simulink model "c28335_pmsmfoc"  (R2021b)
settings: Solver=FixedStepDiscrete  StartTime=0.0  StopTime=0.14  FixedStep=ctrlConst.TsHi  RelTol=1e-3
PreLoadFcn:
  | c28335_pmsmfoc_data
values from neighbouring files (symbols this model uses):
  ctrlConst = struct    [c28335_pmsmfoc_data.m]
  ctrlParams = tmp_P    [c28335_pmsmfoc_data.m]
undefined symbols (not defined in the file or in its folder): DiscIntNeverNeededParam, EnumControllerMode, EnumErrorType
libraries: simulink x11, slpidlib x4
(part 2 of 2)

== system c28335_pmsmfoc/Motor_Control/Field_Oriented_Controller/Current_Control/Transform_Coordinates_ABC_to_dq/Clarke_Transform ==
  note: Clarke Transform
  note: Converts balanced three-phase quantities into balanced two-phase quantities.
      | The A and B phases are converted to the direct axis (alpha) component and the quadrature axis (beta) component.
      | The alpha and beta components are still dependent on time and speed.
  phase_currents : Inport
  A_phase_current : Selector  InputPortWidth=2  IndexOptions=Index vector (dialog)  Indices=1  OutputSizes=1
  Add : Sum
  B_Gain : Gain  Gain=2
  B_phase_current : Selector  InputPortWidth=2  IndexOptions=Index vector (dialog)  Indices=2  OutputSizes=1
  Beta_Gain : Gain  Gain=1/sqrt(3)
  alpha_current : Outport
  beta_current : Outport  Port=2
  wires:
  B_phase_current/1 -> B_Gain/1
  B_Gain/1 -> Add/2
  Add/1 -> Beta_Gain/1
  Beta_Gain/1 -> beta_current/1
  phase_currents/1 -> A_phase_current/1, B_phase_current/1
  A_phase_current/1 -> Add/1, alpha_current/1

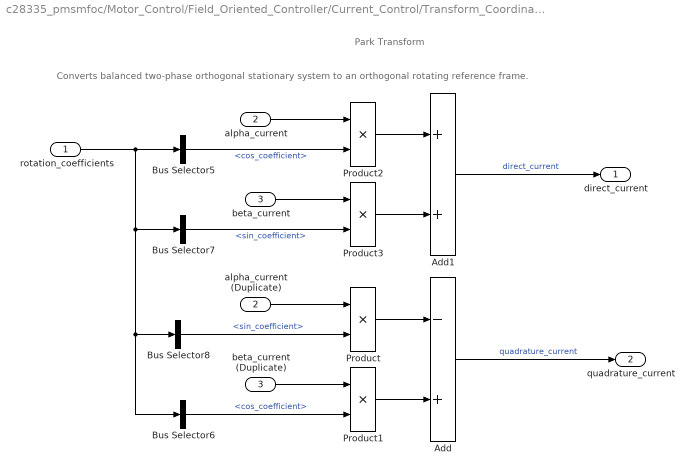
== system c28335_pmsmfoc/Motor_Control/Field_Oriented_Controller/Current_Control/Transform_Coordinates_ABC_to_dq/Park_Transform ==
  note: Park Transform
  note: Converts balanced two-phase orthogonal stationary system to an orthogonal rotating reference frame.
  rotation_coefficients : Inport
  alpha_current : Inport  Port=2
  beta_current : Inport  Port=3
  Add : Sum  Inputs=-+
  Add1 : Sum
  Bus Selector5 : BusSelector  OutputSignals=cos_coefficient
  Bus Selector6 : BusSelector  OutputSignals=cos_coefficient
  Bus Selector7 : BusSelector  OutputSignals=sin_coefficient
  Bus Selector8 : BusSelector  OutputSignals=sin_coefficient
  Product{,1..3} (4 alike) : Product  RndMeth=Zero
  alpha_current (Duplicate) : InportShadow  Port=2
  beta_current (Duplicate) : InportShadow  Port=3
  direct_current : Outport
  quadrature_current : Outport  Port=2
  wires:
  Product/1 -> Add/1
  Product1/1 -> Add/2
  Add/1 -> quadrature_current/1  "quadrature_current"
  Product2/1 -> Add1/1
  Product3/1 -> Add1/2
  Add1/1 -> direct_current/1  "direct_current"
  alpha_current (Duplicate)/1 -> Product/1
  Bus Selector8/1 -> Product/2  "<sin_coefficient>"
  Bus Selector6/1 -> Product1/2  "<cos_coefficient>"
  beta_current (Duplicate)/1 -> Product1/1
  alpha_current/1 -> Product2/1
  Bus Selector5/1 -> Product2/2  "<cos_coefficient>"
  beta_current/1 -> Product3/1
  Bus Selector7/1 -> Product3/2  "<sin_coefficient>"
  rotation_coefficients/1 -> Bus Selector5/1, Bus Selector7/1, Bus Selector8/1, Bus Selector6/1

== system c28335_pmsmfoc/Motor_Control/Field_Oriented_Controller/Current_Control/Transform_Coordinates_dq_to_ABC/Alpha_Beta_to_ABC ==
  note: 1) Only subsystems can be added as variant choices at this level
      | 2) Blocks cannot be connected at this level as connectivity is
      | automatically determined at simulation, based on the active variant
  note: Specifies which Alpha Beta to ABC coordinate transform to use.
      | The Inverse Clarke Transform is a direct sinusoidal coordinate transformation.
      | Space Vector Modulation is a technique to achieve an additional 15% increase in relative voltages between phases.
  note: Alpha Beta to ABC (Variant Subsystem)
  alpha_voltage : Inport
  beta_voltage : Inport  Port=2
  Inverse_Clarke_Transform : Subsystem  VariantControl=INVERSE_CLARKE_TRANSFORM
  Space_Vector_Modulation : Subsystem  VariantControl=SPACE_VECTOR_MODULATION
  phase_voltages : Outport

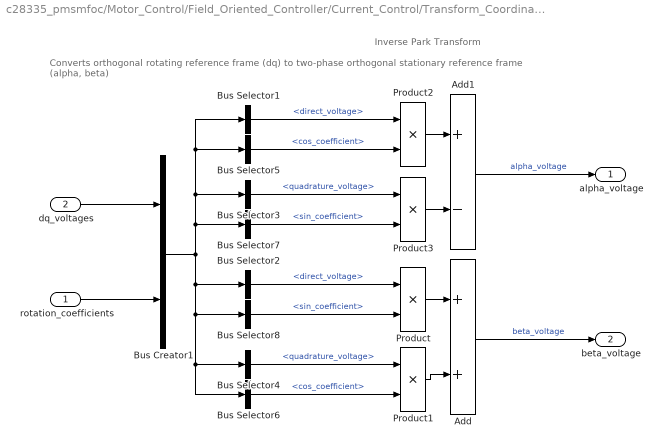
== system c28335_pmsmfoc/Motor_Control/Field_Oriented_Controller/Current_Control/Transform_Coordinates_dq_to_ABC/Inverse_Park_Transform ==
  note: Inverse Park Transform
  note: Converts orthogonal rotating reference frame (dq) to two-phase orthogonal stationary reference frame (alpha, beta)
  rotation_coefficients : Inport
  dq_voltages : Inport  Port=2
  Add : Sum
  Add1 : Sum  Inputs=+-
  Bus Creator1 : BusCreator  Inputs=2
  Bus Selector1 : BusSelector  OutputSignals=signal1.direct_voltage
  Bus Selector2 : BusSelector  OutputSignals=signal1.direct_voltage
  Bus Selector3 : BusSelector  OutputSignals=signal1.quadrature_voltage
  Bus Selector4 : BusSelector  OutputSignals=signal1.quadrature_voltage
  Bus Selector5 : BusSelector  OutputSignals=signal2.cos_coefficient
  Bus Selector6 : BusSelector  OutputSignals=signal2.cos_coefficient
  Bus Selector7 : BusSelector  OutputSignals=signal2.sin_coefficient
  Bus Selector8 : BusSelector  OutputSignals=signal2.sin_coefficient
  Product{,1..3} (4 alike) : Product  RndMeth=Zero
  alpha_voltage : Outport
  beta_voltage : Outport  Port=2
  wires:
  Product/1 -> Add/1
  Product1/1 -> Add/2
  Add/1 -> beta_voltage/1  "beta_voltage"
  Product2/1 -> Add1/1
  Product3/1 -> Add1/2
  Add1/1 -> alpha_voltage/1  "alpha_voltage"
  Bus Selector2/1 -> Product/1  "<direct_voltage>"
  Bus Selector8/1 -> Product/2  "<sin_coefficient>"
  Bus Selector6/1 -> Product1/2  "<cos_coefficient>"
  Bus Selector4/1 -> Product1/1  "<quadrature_voltage>"
  Bus Selector5/1 -> Product2/2  "<cos_coefficient>"
  Bus Selector3/1 -> Product3/1  "<quadrature_voltage>"
  Bus Selector7/1 -> Product3/2  "<sin_coefficient>"
  dq_voltages/1 -> Bus Creator1/1
  rotation_coefficients/1 -> Bus Creator1/2
  Bus Selector1/1 -> Product2/1  "<direct_voltage>"
  Bus Creator1/1 -> Bus Selector1/1, Bus Selector5/1, Bus Selector3/1, Bus Selector7/1, Bus Selector2/1, Bus Selector8/1, Bus Selector4/1, Bus Selector6/1

== system c28335_pmsmfoc/Motor_Control/Sensors_To_Engineering_Units/Position_To_Velocity/Explicit_Angle_Wrap_With_Error/Detect_Velocity_Error ==
  note: Detect Velocity Change Error
  note: If the controller is in VelocityControl mode and the velocity changes more than a realistic amount
      | then generate an error.
  V : Inport
  M : Inport  Port=2
  AND : Logic  AllPortsSameDT=off  OutDataTypeStr=boolean
  Enumerated_Constant : simulink/Sources/Enumerated Constant  OutDataTypeStr=Enum: EnumControllerMode  Value=EnumControllerMode.VelocityControl  SampleTime=inf
  Excessive_Velocity_Change : RelationalOperator  OutDataTypeStr=boolean  RndMeth=Nearest
  Generate_Error : Subsystem  TreatAsAtomicUnit=on
  Max_Valid_Velocity_Change : Constant  Value=pi/ctrlConst.TsLo  OutDataTypeStr=single
  Relational_Operator : RelationalOperator  Operator===  OutDataTypeStr=boolean  RndMeth=Nearest
  Velocity_Abs : Abs
  Velocity_Delay : Delay  DelayLength=1
  Velocity_Difference : Sum  Inputs=+-
  wires:
  Velocity_Abs/1 -> Excessive_Velocity_Change/1
  Max_Valid_Velocity_Change/1 -> Excessive_Velocity_Change/2
  Velocity_Difference/1 -> Velocity_Abs/1
  Velocity_Delay/1 -> Velocity_Difference/2
  V/1 -> Velocity_Difference/1, Velocity_Delay/1  "velocity"
  M/1 -> Relational_Operator/1  "controller_mode"
  Enumerated_Constant/1 -> Relational_Operator/2
  Excessive_Velocity_Change/1 -> AND/2
  Relational_Operator/1 -> AND/1
  AND/1 -> Generate_Error/Enable

== system c28335_pmsmfoc/Motor_Control/Sensors_To_Engineering_Units/Position_To_Velocity/Implicit_Integer_Wrap_With_Error/Detect_Velocity_Error ==
  note: Detect Velocity Change Error
  note: If the controller is in VelocityControl mode and the velocity changes more than a realistic amount
      | then generate an error.
  V : Inport
  M : Inport  Port=2
  AND : Logic  AllPortsSameDT=off  OutDataTypeStr=boolean
  Enumerated_Constant : simulink/Sources/Enumerated Constant  OutDataTypeStr=Enum: EnumControllerMode  Value=EnumControllerMode.VelocityControl  SampleTime=inf
  Excessive_Velocity_Change : RelationalOperator  OutDataTypeStr=boolean  RndMeth=Nearest
  Generate_Error : Subsystem  TreatAsAtomicUnit=on
  Max_Valid_Velocity_Change : Constant  Value=pi/ctrlConst.TsLo  OutDataTypeStr=single
  Relational_Operator : RelationalOperator  Operator===  OutDataTypeStr=boolean  RndMeth=Nearest
  Velocity_Abs : Abs
  Velocity_Delay : Delay  DelayLength=1
  Velocity_Difference : Sum  Inputs=+-
  wires:
  Velocity_Abs/1 -> Excessive_Velocity_Change/1
  Max_Valid_Velocity_Change/1 -> Excessive_Velocity_Change/2
  Velocity_Difference/1 -> Velocity_Abs/1
  Velocity_Delay/1 -> Velocity_Difference/2
  V/1 -> Velocity_Difference/1, Velocity_Delay/1  "velocity"
  M/1 -> Relational_Operator/1  "controller_mode"
  Enumerated_Constant/1 -> Relational_Operator/2
  Excessive_Velocity_Change/1 -> AND/2
  Relational_Operator/1 -> AND/1
  AND/1 -> Generate_Error/Enable

== system c28335_pmsmfoc/Motor_Control/Field_Oriented_Controller/Current_Control/Transform_Coordinates_dq_to_ABC/Alpha_Beta_to_ABC/Inverse_Clarke_Transform ==
  note: Inverse Clarke Transform
  note: Converts direct axis (alpha) component and the quadrature axis (beta) component to balanced three-phase quantities
      | The alpha and beta components are dependent on time and speed.
  alpha_voltage : Inport
  beta_voltage : Inport  Port=2
  Add : Sum  Inputs=-+
  Add1 : Sum  Inputs=--
  Add2 : Sum
  Gain : Gain  Gain=1/2
  Gain1 : Gain  Gain=sqrt(3)/2
  Half_Bus_Voltage : Constant  Value=ctrlConst.BusVoltage/2  OutDataTypeStr=single
  Mux : Mux  Inputs=3
  Signal Conversion : SignalConversion  OverrideOpt=off
  phase_voltages : Outport
  wires:
  Gain/1 -> Add1/1, Add/1
  Gain1/1 -> Add1/2, Add/2
  Add/1 -> Mux/2  "voltage_phase_b"
  Add1/1 -> Mux/3  "voltage_phase_c"
  beta_voltage/1 -> Gain1/1
  alpha_voltage/1 -> Gain/1, Signal Conversion/1
  Mux/1 -> Add2/1
  Add2/1 -> phase_voltages/1
  Half_Bus_Voltage/1 -> Add2/2
  Signal Conversion/1 -> Mux/1  "voltage_phase_a"

== system c28335_pmsmfoc/Motor_Control/Field_Oriented_Controller/Current_Control/Transform_Coordinates_dq_to_ABC/Alpha_Beta_to_ABC/Space_Vector_Modulation ==
  note: Space Vector Modulation
  note: Calculates stator phase voltages using a switching sequence scheme which results in three pseudo-sinusoidal currents in the stator phases.
      | This technique approximates a given stator reference voltage vector by combining the switching pattern corresponding to the basic space vectors.
  alpha_voltage : Inport
  beta_voltage : Inport  Port=2
  Calculate_Phase_Voltages : Subsystem
  Determine_Sector : Subsystem
  Phase_Advanced_Inverse_Clarke : Subsystem
  alpha_voltage (Duplicate) : InportShadow
  beta_voltage (Duplicate) : InportShadow  Port=2
  phase_voltages : Outport
  wires:
  Calculate_Phase_Voltages/1(phase_voltages) -> phase_voltages/1
  Determine_Sector/1(sector) -> Calculate_Phase_Voltages/1(Sector)
  Phase_Advanced_Inverse_Clarke/1(" VA") -> Determine_Sector/1(VA)
  Phase_Advanced_Inverse_Clarke/2(VB) -> Determine_Sector/2(VB)
  Phase_Advanced_Inverse_Clarke/3(VC) -> Determine_Sector/3(VC)
  beta_voltage (Duplicate)/1 -> Calculate_Phase_Voltages/3(beta_voltage)
  alpha_voltage (Duplicate)/1 -> Calculate_Phase_Voltages/2(alpha_voltage)
  alpha_voltage/1 -> Phase_Advanced_Inverse_Clarke/1(alpha_voltage)
  beta_voltage/1 -> Phase_Advanced_Inverse_Clarke/2(beta_voltage)

== system c28335_pmsmfoc/Motor_Control/Sensors_To_Engineering_Units/Position_To_Velocity/Explicit_Angle_Wrap_With_Error/Detect_Velocity_Error/Generate_Error ==
  note: Generate Error
  Enable : EnablePort
  Data_Store_Write : DataStoreWrite  DataStoreName=error  IndexOptions=Index vector (dialog)  Indices=1  OutputSizes=1
  Enumerated_Constant : simulink/Sources/Enumerated Constant  OutDataTypeStr=Enum: EnumErrorType  Value=EnumErrorType.MeasuredVelocityError  SampleTime=inf
  wires:
  Enumerated_Constant/1 -> Data_Store_Write/1

== system c28335_pmsmfoc/Motor_Control/Sensors_To_Engineering_Units/Position_To_Velocity/Implicit_Integer_Wrap_With_Error/Detect_Velocity_Error/Generate_Error ==
  note: Generate Error
  Enable : EnablePort
  Data_Store_Write : DataStoreWrite  DataStoreName=error  IndexOptions=Index vector (dialog)  Indices=1  OutputSizes=1
  Enumerated_Constant : simulink/Sources/Enumerated Constant  OutDataTypeStr=Enum: EnumErrorType  Value=EnumErrorType.MeasuredVelocityError  SampleTime=inf
  wires:
  Enumerated_Constant/1 -> Data_Store_Write/1

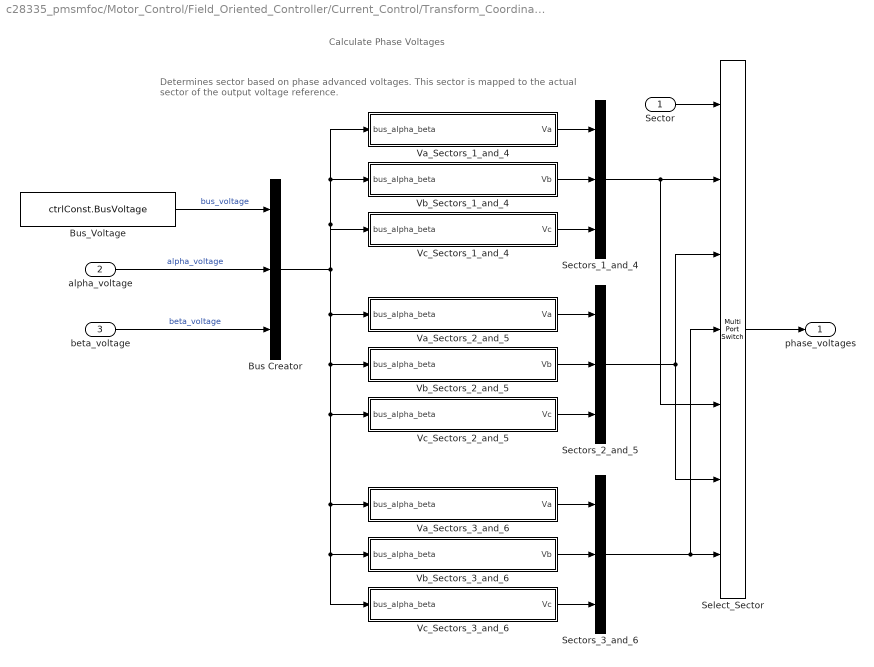
== system c28335_pmsmfoc/Motor_Control/Field_Oriented_Controller/Current_Control/Transform_Coordinates_dq_to_ABC/Alpha_Beta_to_ABC/Space_Vector_Modulation/Calculate_Phase_Voltages ==
  note: Calculate Phase Voltages
  note: Determines sector based on phase advanced voltages.
      | This sector is mapped to the actual sector of the output voltage reference.
  Sector : Inport
  alpha_voltage : Inport  Port=2
  beta_voltage : Inport  Port=3
  Bus Creator : BusCreator  Inputs=3
  Bus_Voltage : Constant  Value=ctrlConst.BusVoltage  OutDataTypeStr=single
  Sectors_1_and_4 : Concatenate  NumInputs=3
  Sectors_2_and_5 : Concatenate  NumInputs=3
  Sectors_3_and_6 : Concatenate  NumInputs=3
  Select_Sector : MultiPortSwitch  Inputs=6
  Va_Sectors_1_and_4 : Subsystem
  Va_Sectors_2_and_5 : Subsystem
  Va_Sectors_3_and_6 : Subsystem
  Vb_Sectors_1_and_4 : Subsystem
  Vb_Sectors_2_and_5 : Subsystem
  Vb_Sectors_3_and_6 : Subsystem
  Vc_Sectors_1_and_4 : Subsystem
  Vc_Sectors_2_and_5 : Subsystem
  Vc_Sectors_3_and_6 : Subsystem
  phase_voltages : Outport
  wires:
  Sector/1 -> Select_Sector/1
  Bus Creator/1 -> Va_Sectors_1_and_4/1(bus_alpha_beta), Vb_Sectors_1_and_4/1(bus_alpha_beta), Vc_Sectors_1_and_4/1(bus_alpha_beta), Va_Sectors_2_and_5/1(bus_alpha_beta), Vb_Sectors_2_and_5/1(bus_alpha_beta), Vc_Sectors_2_and_5/1(bus_alpha_beta), Va_Sectors_3_and_6/1(bus_alpha_beta), Vb_Sectors_3_and_6/1(bus_alpha_beta), Vc_Sectors_3_and_6/1(bus_alpha_beta)
  Va_Sectors_1_and_4/1(Va) -> Sectors_1_and_4/1
  Vb_Sectors_1_and_4/1(Vb) -> Sectors_1_and_4/2
  Vc_Sectors_1_and_4/1(Vc) -> Sectors_1_and_4/3
  Va_Sectors_2_and_5/1(Va) -> Sectors_2_and_5/1
  Vb_Sectors_2_and_5/1(Vb) -> Sectors_2_and_5/2
  Vc_Sectors_2_and_5/1(Vc) -> Sectors_2_and_5/3
  Va_Sectors_3_and_6/1(Va) -> Sectors_3_and_6/1
  Vb_Sectors_3_and_6/1(Vb) -> Sectors_3_and_6/2
  Vc_Sectors_3_and_6/1(Vc) -> Sectors_3_and_6/3
  Sectors_1_and_4/1 -> Select_Sector/2, Select_Sector/5
  Sectors_2_and_5/1 -> Select_Sector/3, Select_Sector/6
  Sectors_3_and_6/1 -> Select_Sector/7, Select_Sector/4
  Select_Sector/1 -> phase_voltages/1
  Bus_Voltage/1 -> Bus Creator/1  "bus_voltage"
  alpha_voltage/1 -> Bus Creator/2  "alpha_voltage"
  beta_voltage/1 -> Bus Creator/3  "beta_voltage"

== system c28335_pmsmfoc/Motor_Control/Field_Oriented_Controller/Current_Control/Transform_Coordinates_dq_to_ABC/Alpha_Beta_to_ABC/Space_Vector_Modulation/Determine_Sector ==
  note: Determine Sector
  note: Determines sector based on phase advanced voltages.
      | This sector is mapped to the actual sector of the output voltage reference.
  VA : Inport
  VB : Inport  Port=2
  VC : Inport  Port=3
  Calculate_Phase_Advanced_Sector : Sum  Inputs=+++
  Compare_VA_To_Zero : simulink/Logic and Bit Operations/Compare To Zero  relop=>  OutDataTypeStr=uint8
  Compare_VB_To_Zero : simulink/Logic and Bit Operations/Compare To Zero  relop=>  OutDataTypeStr=uint8
  Compare_VC_To_Zero : simulink/Logic and Bit Operations/Compare To Zero  relop=>  OutDataTypeStr=uint8
  Lookup_Table : LookupNDDirect  NumberOfTableDimensions=1  Table=[2,2,6,1,4,3,5]  TableDataTypeStr=uint16
      settings: AttributesFormatString=-------------------------------\nTable: %<Table>
  Sector_Gain_VB : Gain  Gain=2  ParamDataTypeStr=int16  OutDataTypeStr=int16
  Sector_Gain_VC : Gain  Gain=4  ParamDataTypeStr=int16  OutDataTypeStr=int16
  sector : Outport
  wires:
  Compare_VA_To_Zero/1 -> Calculate_Phase_Advanced_Sector/1
  Compare_VB_To_Zero/1 -> Sector_Gain_VB/1
  Sector_Gain_VB/1 -> Calculate_Phase_Advanced_Sector/2
  Compare_VC_To_Zero/1 -> Sector_Gain_VC/1
  Sector_Gain_VC/1 -> Calculate_Phase_Advanced_Sector/3
  VA/1 -> Compare_VA_To_Zero/1
  VB/1 -> Compare_VB_To_Zero/1
  VC/1 -> Compare_VC_To_Zero/1
  Lookup_Table/1 -> sector/1
  Calculate_Phase_Advanced_Sector/1 -> Lookup_Table/1

== system c28335_pmsmfoc/Motor_Control/Field_Oriented_Controller/Current_Control/Transform_Coordinates_dq_to_ABC/Alpha_Beta_to_ABC/Space_Vector_Modulation/Phase_Advanced_Inverse_Clarke ==
  note: Phase Advanced Inverse Clarke Transform
  note: Projects the quadrature (beta) component (as opposed to the conventional inverse Clarke transform
      | which projects the alpha component).
  alpha_voltage : Inport
  beta_voltage : Inport  Port=2
  Add : Sum  Inputs=-+
  Add1 : Sum  Inputs=--
  Gain : Gain  Gain=1/2
  Gain1 : Gain  Gain=sqrt(3)/2
  " VA" : Outport
  VB : Outport  Port=2
  VC : Outport  Port=3
  wires:
  Gain/1 -> Add1/1, Add/1
  alpha_voltage/1 -> Gain1/1
  Gain1/1 -> Add1/2, Add/2
  Add/1 -> VB/1  "voltage_phase_b"
  Add1/1 -> VC/1  "voltage_phase_c"
  beta_voltage/1 -> Gain/1, " VA"/1

== system c28335_pmsmfoc/Motor_Control/Field_Oriented_Controller/Current_Control/Transform_Coordinates_dq_to_ABC/Alpha_Beta_to_ABC/Space_Vector_Modulation/Calculate_Phase_Voltages/Va_Sectors_1_and_4 ==
  note: Va Sectors 1 and 4
  note: Calculate space vector voltage
  bus_alpha_beta : Inport
  Add : Sum  Inputs=+++
  Alpha_Gain : Gain  Gain=sqrt(3)
  Bus Selector : BusSelector  OutputSignals=bus_voltage,alpha_voltage,beta_voltage
  Bus_Gain : Gain  Gain=sqrt(2)
  Space_Vector_Gain : Gain  Gain=sqrt(2)/4
  Va : Outport
  wires:
  Bus Selector/1 -> Bus_Gain/1  "<bus_voltage>"
  Bus_Gain/1 -> Add/1
  Alpha_Gain/1 -> Add/2
  Add/1 -> Space_Vector_Gain/1
  Space_Vector_Gain/1 -> Va/1
  Bus Selector/2 -> Alpha_Gain/1  "<alpha_voltage>"
  Bus Selector/3 -> Add/3  "<beta_voltage>"
  bus_alpha_beta/1 -> Bus Selector/1

== system c28335_pmsmfoc/Motor_Control/Field_Oriented_Controller/Current_Control/Transform_Coordinates_dq_to_ABC/Alpha_Beta_to_ABC/Space_Vector_Modulation/Calculate_Phase_Voltages/Va_Sectors_2_and_5 ==
  note: Calculate space vector voltage
  note: Va Sectors 2 and 5
  bus_alpha_beta : Inport
  Add : Sum
  Alpha_Gain : Gain  Gain=sqrt(6)
  Bus Selector : BusSelector  OutputSignals=bus_voltage,alpha_voltage
  Space_Vector_Gain : Gain  Gain=1/2
  Va : Outport
  wires:
  bus_alpha_beta/1 -> Bus Selector/1
  Bus Selector/2 -> Alpha_Gain/1  "<alpha_voltage>"
  Space_Vector_Gain/1 -> Va/1
  Add/1 -> Space_Vector_Gain/1
  Alpha_Gain/1 -> Add/2
  Bus Selector/1 -> Add/1  "<bus_voltage>"

== system c28335_pmsmfoc/Motor_Control/Field_Oriented_Controller/Current_Control/Transform_Coordinates_dq_to_ABC/Alpha_Beta_to_ABC/Space_Vector_Modulation/Calculate_Phase_Voltages/Va_Sectors_3_and_6 ==
  note: Va Sectors 3 and 6
  note: Calculate space vector voltage
  bus_alpha_beta : Inport
  Add : Sum  Inputs=++-
  Alpha_Gain : Gain  Gain=sqrt(3)
  Bus Selector : BusSelector  OutputSignals=bus_voltage,alpha_voltage,beta_voltage
  Bus_Gain : Gain  Gain=sqrt(2)
  Space_Vector_Gain : Gain  Gain=sqrt(2)/4
  Va : Outport
  wires:
  Bus Selector/1 -> Bus_Gain/1  "<bus_voltage>"
  Bus_Gain/1 -> Add/1
  Alpha_Gain/1 -> Add/2
  Add/1 -> Space_Vector_Gain/1
  Space_Vector_Gain/1 -> Va/1
  Bus Selector/2 -> Alpha_Gain/1  "<alpha_voltage>"
  Bus Selector/3 -> Add/3  "<beta_voltage>"
  bus_alpha_beta/1 -> Bus Selector/1

== system c28335_pmsmfoc/Motor_Control/Field_Oriented_Controller/Current_Control/Transform_Coordinates_dq_to_ABC/Alpha_Beta_to_ABC/Space_Vector_Modulation/Calculate_Phase_Voltages/Vb_Sectors_1_and_4 ==
  note: Calculate space vector voltage
  note: Vb Sectors 1 and 4
  bus_alpha_beta : Inport
  Add : Sum  Inputs=+-+
  Alpha_Gain : Gain  Gain=sqrt(3)
  Beta_Gain : Gain  Gain=3
  Bus Selector : BusSelector  OutputSignals=bus_voltage,alpha_voltage,beta_voltage
  Bus_Gain : Gain  Gain=sqrt(2)
  Va_Gain : Gain  Gain=sqrt(2)/4
  Vb : Outport
  wires:
  bus_alpha_beta/1 -> Bus Selector/1
  Bus Selector/3 -> Beta_Gain/1  "<beta_voltage>"
  Bus Selector/2 -> Alpha_Gain/1  "<alpha_voltage>"
  Va_Gain/1 -> Vb/1
  Add/1 -> Va_Gain/1
  Beta_Gain/1 -> Add/3
  Alpha_Gain/1 -> Add/2
  Bus_Gain/1 -> Add/1
  Bus Selector/1 -> Bus_Gain/1  "<bus_voltage>"

== system c28335_pmsmfoc/Motor_Control/Field_Oriented_Controller/Current_Control/Transform_Coordinates_dq_to_ABC/Alpha_Beta_to_ABC/Space_Vector_Modulation/Calculate_Phase_Voltages/Vb_Sectors_2_and_5 ==
  note: Vb Sectors 2 and 5
  note: Calculate space vector voltage
  bus_alpha_beta : Inport
  Add : Sum
  Beta_Gain : Gain  Gain=sqrt(2)
  Bus Selector : BusSelector  OutputSignals=bus_voltage,beta_voltage
  Va_Gain : Gain  Gain=1/2
  Vb : Outport
  wires:
  Bus Selector/1 -> Add/1  "<bus_voltage>"
  Beta_Gain/1 -> Add/2
  Add/1 -> Va_Gain/1
  Va_Gain/1 -> Vb/1
  Bus Selector/2 -> Beta_Gain/1  "<beta_voltage>"
  bus_alpha_beta/1 -> Bus Selector/1

== system c28335_pmsmfoc/Motor_Control/Field_Oriented_Controller/Current_Control/Transform_Coordinates_dq_to_ABC/Alpha_Beta_to_ABC/Space_Vector_Modulation/Calculate_Phase_Voltages/Vb_Sectors_3_and_6 ==
  note: Calculate space vector voltage
  note: Vb Sectors 3 and 6
  bus_alpha_beta : Inport
  Add : Sum  Inputs=+-+
  Alpha_Gain : Gain  Gain=sqrt(3)
  Bus Selector : BusSelector  OutputSignals=bus_voltage,alpha_voltage,beta_voltage
  Bus_Gain : Gain  Gain=sqrt(2)
  Va_Gain : Gain  Gain=sqrt(2)/4
  Vb : Outport
  wires:
  bus_alpha_beta/1 -> Bus Selector/1
  Bus Selector/3 -> Add/3  "<beta_voltage>"
  Bus Selector/2 -> Alpha_Gain/1  "<alpha_voltage>"
  Va_Gain/1 -> Vb/1
  Add/1 -> Va_Gain/1
  Alpha_Gain/1 -> Add/2
  Bus_Gain/1 -> Add/1
  Bus Selector/1 -> Bus_Gain/1  "<bus_voltage>"

== system c28335_pmsmfoc/Motor_Control/Field_Oriented_Controller/Current_Control/Transform_Coordinates_dq_to_ABC/Alpha_Beta_to_ABC/Space_Vector_Modulation/Calculate_Phase_Voltages/Vc_Sectors_1_and_4 ==
  note: Vc Sectors 1 and 4
  note: Calculate space vector voltage
  bus_alpha_beta : Inport
  Add : Sum  Inputs=+--
  Alpha_Gain : Gain  Gain=sqrt(3)
  Bus Selector : BusSelector  OutputSignals=bus_voltage,alpha_voltage,beta_voltage
  Bus_Gain : Gain  Gain=sqrt(2)
  Space_Vector_Gain : Gain  Gain=sqrt(2)/4
  Vc : Outport
  wires:
  Bus Selector/1 -> Bus_Gain/1  "<bus_voltage>"
  Bus_Gain/1 -> Add/1
  Alpha_Gain/1 -> Add/2
  Add/1 -> Space_Vector_Gain/1
  Space_Vector_Gain/1 -> Vc/1
  Bus Selector/2 -> Alpha_Gain/1  "<alpha_voltage>"
  Bus Selector/3 -> Add/3  "<beta_voltage>"
  bus_alpha_beta/1 -> Bus Selector/1

== system c28335_pmsmfoc/Motor_Control/Field_Oriented_Controller/Current_Control/Transform_Coordinates_dq_to_ABC/Alpha_Beta_to_ABC/Space_Vector_Modulation/Calculate_Phase_Voltages/Vc_Sectors_2_and_5 ==
  note: Calculate space vector voltage
  note: Vc Sectors 2 and 5
  bus_alpha_beta : Inport
  Add : Sum  Inputs=+-
  Beta_Gain : Gain  Gain=sqrt(2)
  Bus Selector : BusSelector  OutputSignals=bus_voltage,beta_voltage
  Space_Vector_Gain : Gain  Gain=1/2
  Vc : Outport
  wires:
  bus_alpha_beta/1 -> Bus Selector/1
  Bus Selector/2 -> Beta_Gain/1  "<beta_voltage>"
  Space_Vector_Gain/1 -> Vc/1
  Add/1 -> Space_Vector_Gain/1
  Beta_Gain/1 -> Add/2
  Bus Selector/1 -> Add/1  "<bus_voltage>"

== system c28335_pmsmfoc/Motor_Control/Field_Oriented_Controller/Current_Control/Transform_Coordinates_dq_to_ABC/Alpha_Beta_to_ABC/Space_Vector_Modulation/Calculate_Phase_Voltages/Vc_Sectors_3_and_6 ==
  note: Vc Sectors 3 and 6
  note: Calculate space vector voltage
  bus_alpha_beta : Inport
  Add : Sum  Inputs=+--
  Alpha_Gain : Gain  Gain=sqrt(3)
  Beta_Gain : Gain  Gain=3
  Bus Selector : BusSelector  OutputSignals=bus_voltage,alpha_voltage,beta_voltage
  Bus_Gain : Gain  Gain=sqrt(2)
  Space_Vector_Gain : Gain  Gain=sqrt(2)/4
  Vc : Outport
  wires:
  Bus Selector/1 -> Bus_Gain/1  "<bus_voltage>"
  Bus_Gain/1 -> Add/1
  Alpha_Gain/1 -> Add/2
  Beta_Gain/1 -> Add/3
  Add/1 -> Space_Vector_Gain/1
  Space_Vector_Gain/1 -> Vc/1
  Bus Selector/2 -> Alpha_Gain/1  "<alpha_voltage>"
  Bus Selector/3 -> Beta_Gain/1  "<beta_voltage>"
  bus_alpha_beta/1 -> Bus Selector/1

== stateflow chart c28335_pmsmfoc/Mode_Scheduler/Controller_Mode_Scheduler ==
  settings: updateMethod=DISCRETE  sampleTime=ctrlConst.TsLo  executeAtInitialization=1
  note: Controller Mode Scheduler
  note: The motor control algorithm begins in a stand-by mode awaiting a command to turn the motor on. Once this command
      | is issued the motor rotates to identify a known rotor position with valid position. The appropriate closed loop control then begins.
      | Upon a request to stop the motor, the motor will decellerate until zero speed is identified, after which the algorithm returns to the stand-by mode.
  state Motor_On
    state Motor_Control
      state Startup_Open_Loop_Control
        entry: controller_mode = Startup;
        torque_command := ctrlParams.StartupCurrent;
      state Velocity_Control
        entry: controller_mode = VelocityControl;
        en, du:
        velocity_command := command;
      state Position_Control
        entry: controller_mode = PositionControl
        en,du:
        position_command := command;
      state Torque_Control
        entry: controller_mode = TorqueControl;
        en, du:
        torque_command := command;
      (junction 132) -> Startup_Open_Loop_Control [order 1] : [~position_valid]
      (junction 132) -> (junction 135) [order 2]
      Startup_Open_Loop_Control -> (junction 135) : [position_valid]
      (junction 135) -> (junction 232)
      (junction 232) -> Velocity_Control [order 1] : [command_type==Velocity]
      (junction 232) -> (junction 159) [order 2]
      (junction 159) -> Position_Control [order 1] : [command_type==Position]
      (junction 159) -> (junction 139) [order 2]
      (junction 139) -> Torque_Control : % [command_type==Torque]
    state Ramp_To_Stop
      entry: controller_mode = VelocityControl;
      velocity_command := 0;
      torque_command := 0;
    Motor_Control -> Ramp_To_Stop : [~motor_on]
  state Stand_By
    entry: controller_mode = StandBy;
  (default) -> Stand_By
  Stand_By -> (junction 132) : [motor_on & ...
      |  ~error]
  (junction 354) -> Stand_By
  (junction 350) -> Stand_By
  Motor_On -> (junction 350) : [error]
  Ramp_To_Stop -> (junction 354) : [abs(velocity) < ...
      | ctrlParams.RampToStopVelocity]
  data: controller_mode output Enum: EnumControllerMode; velocity_command output single; position_valid input; velocity input; motor_on input uint16; position_command output single; command_type input Enum: EnumCommandType; torque_command output single; command input; ctrlParams parameter; error data_store_memory

== stateflow chart c28335_pmsmfoc/Motor_Control/Sensors_To_Engineering_Units/Encoder_To_Position/Wait_For_Valid_Position ==
  settings: updateMethod=DISCRETE
  note: Control Mode Scheduler
  note: Valid absolute position is indicated by an index pulse from the encoder. The velocity signal will be
      | valid after the sample time at which the velocity signal is calculated.
      |
      | If position encoder is valid at first call to function, then go directly to position valid state.
  state Wait_For_Valid_Position
  state Wait_For_Valid_Velocity
  state Position_Valid
  (default) -> (junction 111)
  (junction 111) -> (junction 112) [order 1] : [encoder_valid == 0]
  (junction 111) -> (junction 116) [order 2]
  (junction 112) -> Wait_For_Valid_Position
  Wait_For_Valid_Position -> Wait_For_Valid_Velocity : [encoder_valid]
  Wait_For_Valid_Velocity -> Position_Valid : after(WaitForValidVelocityTicks, tick)
  (junction 116) -> Position_Valid
  data: encoder_valid input; Position_Valid output boolean; WaitForValidVelocityTicks constant int32 =ctrlConst.TsLo/ctrlConst.TsHi
